simulink model "voltage"  (R2023a)
settings: Solver=VariableStepAuto  StartTime=0.0  StopTime=30  RelTol=1e-3
undefined symbols (not defined in the file or in its folder): sigbuilder_block
settings Model: Creator=nineday  LastModifiedBy=nineday
settings ModelReferenceCC: EnableRefExpFcnMdlSchedulingChecks=on

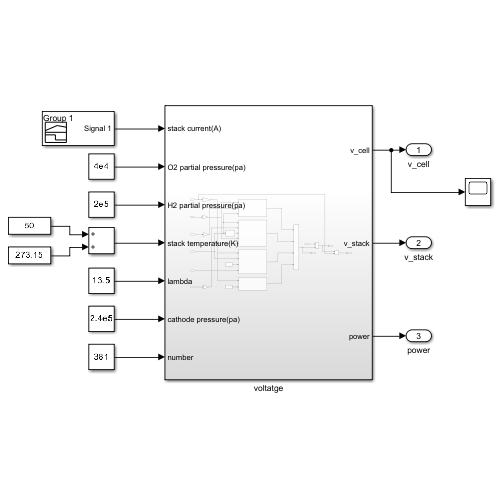
[thumbnail: Simulink's stored preview of the top-level diagram]
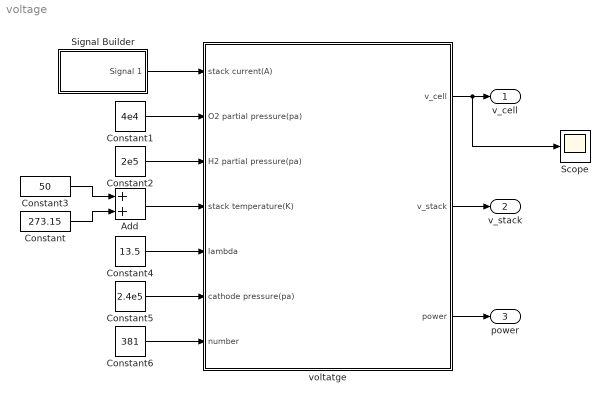
== system voltage ==
  Add : Sum
  Constant : Constant  Value=273.15
  Constant1 : Constant  Value=4e4
  Constant2 : Constant  Value=2e5
  Constant3 : Constant  Value=50
  Constant4 : Constant  Value=13.5
  Constant5 : Constant  Value=2.4e5
  Constant6 : Constant  Value=381
  Scope : Scope
  Signal Builder : Subsystem  Tag=STV Subsys  LoadFcn=sigbuilder_block('load');  StartFcn=sigbuilder_block('start');  StopFcn=sigbuilder_block('stop');  ClipboardFcn=sigbuilder_block('clipboard');  mask(Sigbuilder block){tuvar=[0:10]}
      mask help: Simulink:masks:SigbuilderBlock_MD
      mask init:
      | if ~strcmp(get_param(bdroot(gcbh),'SimulationStatus'),'stopped') tuvar = sigbuilder_block('maskInit'); end
      settings: CopyFcn=sigbuilder_block('copy');  DeleteFcn=sigbuilder_block('delete');  ModelCloseFcn=sigbuilder_block('modelClose');  PreSaveFcn=sigbuilder_block('preSave');  PauseFcn=sigbuilder_block('pause');  ContinueFcn=sigbuilder_block('continue');  NameChangeFcn=sigbuilder_block('namechange');  OpenFcn=sigbuilder_block('open',[591 193.8 786 400.2 ]);  CloseFcn=sigbuilder_block('close');
      mask Display: plot(0, 0, 100, 100,[2, 2, 32, 32, 2], [68, 8, 8, 68, 68],[32, 2], [38, 38], [32, 19, 2],[53, 60, 44], [32, 17, 17, 2],[16, 16, 31, 31]);txt = getActiveGroup(gcbh);text(2, 100, txt,'verticalAlignment', 'top');
  voltatge : Subsystem
  v_cell : Outport
  v_stack : Outport  Port=2
  power : Outport  Port=3
  wires:
  voltatge/3(power) -> power/1
  voltatge/2(v_stack) -> v_stack/1
  voltatge/1(v_cell) -> Scope/1, v_cell/1
  Signal Builder/1(Signal 1) -> voltatge/1(stack current(A))
  Constant6/1 -> voltatge/7(number)
  Constant5/1 -> voltatge/6(cathode pressure(pa))
  Constant4/1 -> voltatge/5(lambda)
  Add/1 -> voltatge/4(stack temperature(K))
  Constant2/1 -> voltatge/3(H2 partial pressure(pa))
  Constant1/1 -> voltatge/2(O2 partial pressure(pa))
  Constant/1 -> Add/2
  Constant3/1 -> Add/1

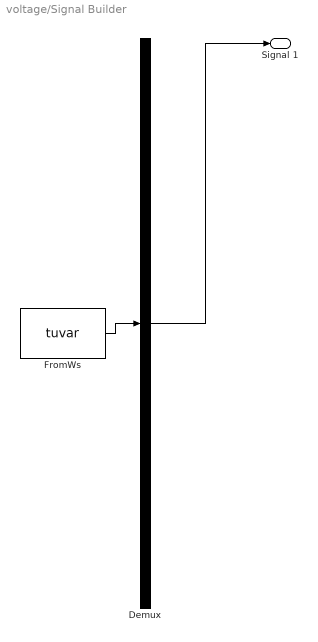
== system voltage/Signal Builder ==
  Demux : Demux  Tag=STV Demux  Outputs=1
      settings: DisplayOption=none
  FromWs : FromWorkspace  Tag=STV FromWs  VariableName=tuvar
      SigBuilderData=|
      | common.afterFinalStr = 'Extrapolate'
      | common.sampleTime = 0
      | dataSet.timeRange = [0 30]
      | dataSet.name = 'Group 1'
      | sbobj.Groups.Name = 'Group 1'
      | sbobj.Groups.Signals.Name = 'Signal 1'
      | sbobj.Groups.Signals.XData = [0 4 6 10 10 30]
      | sbobj.Groups.Signals.YData = [0 4 6 10 10 30]
      | sbobj.Groups.TimeRange = [0 30]
  Signal 1 : Outport  Tag=STV Outport
  wires:
  Demux/1 -> Signal 1/1
  FromWs/1 -> Demux/1

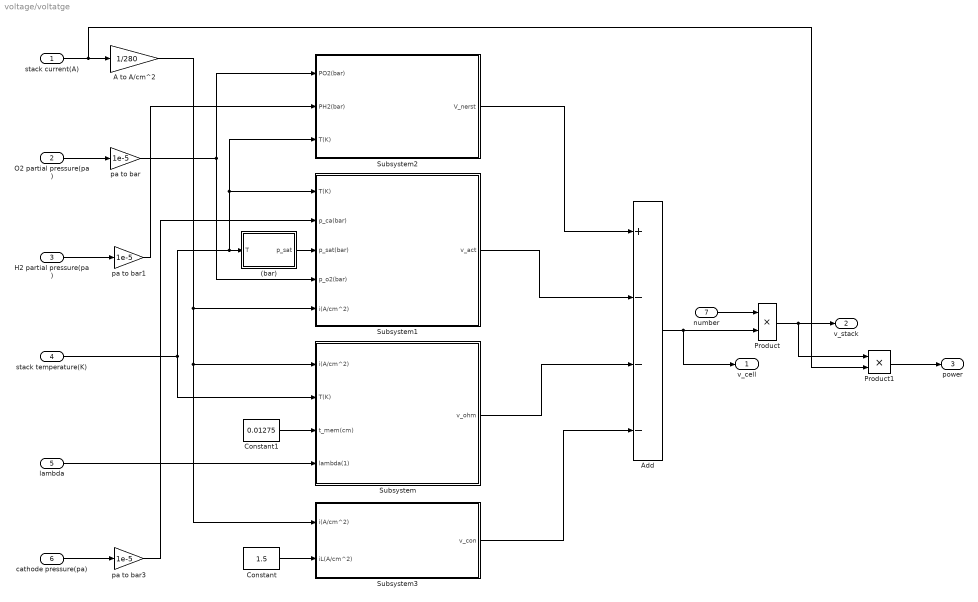
== system voltage/voltatge ==
  stack current(A) : Inport
  O2 partial pressure(pa) : Inport  Port=2
  H2 partial pressure(pa) : Inport  Port=3
  stack temperature(K) : Inport  Port=4
  lambda : Inport  Port=5
  cathode pressure(pa) : Inport  Port=6
  number : Inport  Port=7
  (bar) : MATLAB Function  TreatAsAtomicUnit=on
  A to A/cm^2 : Gain  Gain=1/280
  Add : Sum  Inputs=+---
  Constant : Constant  Value=1.5
  Constant1 : Constant  Value=0.01275
  Product : Product
  Product1 : Product
  Subsystem : Subsystem
  Subsystem1 : Subsystem
  Subsystem2 : Subsystem
  Subsystem3 : Subsystem
  pa to bar : Gain  Gain=1e-5
  pa to bar1 : Gain  Gain=1e-5
  pa to bar3 : Gain  Gain=1e-5
  v_cell : Outport
  v_stack : Outport  Port=2
  power : Outport  Port=3
  wires:
  Add/1 -> v_cell/1, Product/2
  stack temperature(K)/1 -> Subsystem1/1(T(K)), Subsystem2/3(T(K)), (bar)/1(T), Subsystem/2(T(K))
  pa to bar3/1 -> Subsystem1/2(p_ca(bar))
  A to A/cm^2/1 -> Subsystem1/5(i(A/cm^2)), Subsystem3/1(i(A/cm^2)), Subsystem/1(i(A/cm^2))
  Subsystem2/1(V_nerst) -> Add/1
  Subsystem3/1(v_con) -> Add/4
  Subsystem/1(v_ohm) -> Add/3
  H2 partial pressure(pa)/1 -> pa to bar1/1
  (bar)/1(p_sat) -> Subsystem1/3(p_sat(bar))
  pa to bar/1 -> Subsystem2/1(PO2(bar)), Subsystem1/4(p_o2(bar))
  pa to bar1/1 -> Subsystem2/2(PH2(bar))
  number/1 -> Product/1
  O2 partial pressure(pa)/1 -> pa to bar/1
  Constant/1 -> Subsystem3/2(iL(A/cm^2))
  lambda/1 -> Subsystem/4(lambda(1))
  Product1/1 -> power/1
  stack current(A)/1 -> Product1/2, A to A/cm^2/1
  Product/1 -> v_stack/1, Product1/1
  cathode pressure(pa)/1 -> pa to bar3/1
  Constant1/1 -> Subsystem/3(t_mem(cm))
  Subsystem1/1(v_act) -> Add/2

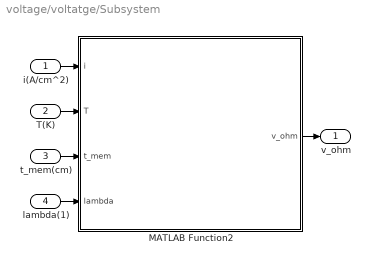
== system voltage/voltatge/Subsystem ==
  i(A/cm^2) : Inport
  T(K) : Inport  Port=2
  t_mem(cm) : Inport  Port=3
  lambda(1) : Inport  Port=4
  MATLAB Function2 : MATLAB Function  TreatAsAtomicUnit=on
  v_ohm : Outport
  wires:
  t_mem(cm)/1 -> MATLAB Function2/3(t_mem)
  MATLAB Function2/1(v_ohm) -> v_ohm/1
  T(K)/1 -> MATLAB Function2/2(T)
  lambda(1)/1 -> MATLAB Function2/4(lambda)
  i(A/cm^2)/1 -> MATLAB Function2/1(i)

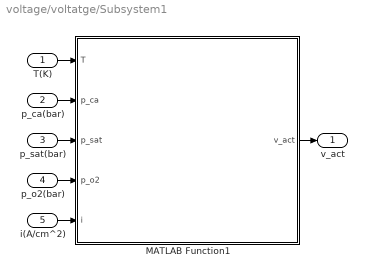
== system voltage/voltatge/Subsystem1 ==
  T(K) : Inport
  p_ca(bar) : Inport  Port=2
  p_sat(bar) : Inport  Port=3
  p_o2(bar) : Inport  Port=4
  i(A/cm^2) : Inport  Port=5
  MATLAB Function1 : MATLAB Function  TreatAsAtomicUnit=on
  v_act : Outport
  wires:
  i(A/cm^2)/1 -> MATLAB Function1/5(i)
  p_ca(bar)/1 -> MATLAB Function1/2(p_ca)
  p_sat(bar)/1 -> MATLAB Function1/3(p_sat)
  T(K)/1 -> MATLAB Function1/1(T)
  MATLAB Function1/1(v_act) -> v_act/1
  p_o2(bar)/1 -> MATLAB Function1/4(p_o2)

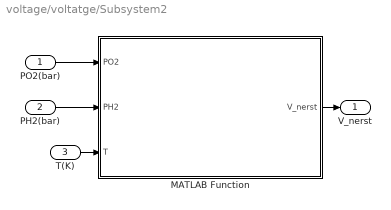
== system voltage/voltatge/Subsystem2 ==
  PO2(bar) : Inport
  PH2(bar) : Inport  Port=2
  T(K) : Inport  Port=3
  MATLAB Function : MATLAB Function  TreatAsAtomicUnit=on
  V_nerst : Outport
  wires:
  PO2(bar)/1 -> MATLAB Function/1(PO2)
  T(K)/1 -> MATLAB Function/3(T)
  MATLAB Function/1(V_nerst) -> V_nerst/1
  PH2(bar)/1 -> MATLAB Function/2(PH2)

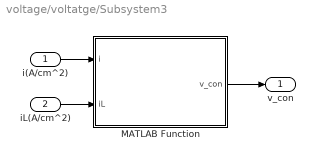
== system voltage/voltatge/Subsystem3 ==
  i(A/cm^2) : Inport
  iL(A/cm^2) : Inport  Port=2
  MATLAB Function : MATLAB Function  TreatAsAtomicUnit=on
  v_con : Outport
  wires:
  iL(A/cm^2)/1 -> MATLAB Function/2(iL)
  i(A/cm^2)/1 -> MATLAB Function/1(i)
  MATLAB Function/1(v_con) -> v_con/1

== matlab function voltage/voltatge/Subsystem1/MATLAB Function1 ==
  data: T input; v_act output; p_ca input; p_sat input; p_o2 input; i input
function v_act = active(T,p_ca,p_sat,p_o2,i)

v0 = 0.279-8.5e-4*(T-298.15)+4.308e-5*T*(log((p_ca-p_sat)/1.01325)+0.5*log(0.1173*(p_ca-p_sat)/1.01325));

va = (-1.618e-5*T + 1.618e-2)*(p_o2/0.1173+p_sat)^2 + (1.8e-4*T-0.166)*(p_o2/0.1173+p_sat) + (-5.8e-4*T+0.5736);

c1 = 10;
v_act = v0 + va*(1-exp(-c1*i));

== matlab function voltage/voltatge/Subsystem2/MATLAB Function ==
  data: PO2 input; PH2 input; T input; V_nerst output
function V_nerst = nerst(PO2,PH2,T )

V_nerst = 1.229-8.5*10^(-4)*(T-298.15)+4.3085*10^(-5)*T*(log(PH2)+0.5*log(PO2));

== matlab function voltage/voltatge/(bar) ==
  data: T input; p_sat output
function p_sat = saturation(T)
p_sat = exp(23.196-3816.44/(T-46.13))*1e-5;

== matlab function voltage/voltatge/Subsystem/MATLAB Function2 ==
  data: i input; T input; v_ohm output; t_mem input; lambda input
function v_ohm = ohm(i, T , t_mem, lambda)

sigma_m = (0.514*lambda - 0.033)*exp(1268*(1/303-1/T));

R_m = t_mem/sigma_m;

R_c = 0;

v_ohm = i*(R_m+R_c);

== matlab function voltage/voltatge/Subsystem3/MATLAB Function ==
  data: i input; v_con output; iL input
function v_con = concentration(i,iL)
B=0.016;
v_con = B*log(iL/(iL-i));
